simulink library "CreateCovDiagMatrix"  (R2018b)
settings: Solver=VariableStepAuto  StartTime=0.0  StopTime=10.0  RelTol=1e-3
settings Model: Creator=BI28030  LastModifiedBy=BI28030

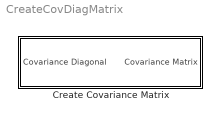
== system CreateCovDiagMatrix ==
  Create Covariance Matrix : Subsystem

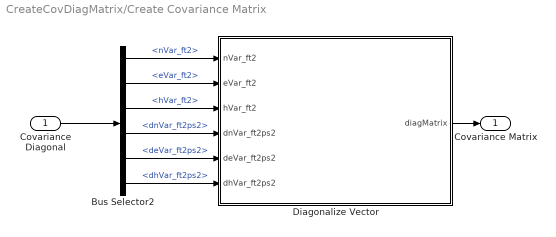
== system CreateCovDiagMatrix/Create Covariance Matrix ==
  Covariance Diagonal : Inport
  Bus Selector2 : BusSelector  OutputSignals=nVar_ft2,eVar_ft2,hVar_ft2,dnVar_ft2ps2,deVar_ft2ps2,dhVar_ft2ps2
  Diagonalize Vector : MATLAB Function  TreatAsAtomicUnit=on
  Covariance Matrix : Outport
  wires:
  Covariance Diagonal/1 -> Bus Selector2/1
  Diagonalize Vector/1(diagMatrix) -> Covariance Matrix/1
  Bus Selector2/1 -> Diagonalize Vector/1(nVar_ft2)  "<nVar_ft2>"
  Bus Selector2/2 -> Diagonalize Vector/2(eVar_ft2)  "<eVar_ft2>"
  Bus Selector2/3 -> Diagonalize Vector/3(hVar_ft2)  "<hVar_ft2>"
  Bus Selector2/4 -> Diagonalize Vector/4(dnVar_ft2ps2)  "<dnVar_ft2ps2>"
  Bus Selector2/5 -> Diagonalize Vector/5(deVar_ft2ps2)  "<deVar_ft2ps2>"
  Bus Selector2/6 -> Diagonalize Vector/6(dhVar_ft2ps2)  "<dhVar_ft2ps2>"

== matlab function CreateCovDiagMatrix/Create Covariance Matrix/Diagonalize Vector ==
  data: nVar_ft2 input; diagMatrix output; eVar_ft2 input; hVar_ft2 input; dnVar_ft2ps2 input; deVar_ft2ps2 input; dhVar_ft2ps2 input
function diagMatrix = createDiagMatrix(nVar_ft2, eVar_ft2, hVar_ft2, dnVar_ft2ps2, deVar_ft2ps2, dhVar_ft2ps2)

diagMatrix = zeros(6);

% diagMatrix(1,1) = diagVector(1);
% diagMatrix(2,2) = diagVector(2);
% diagMatrix(3,3) = diagVector(3);
% diagMatrix(4,4) = diagVector(4);
% diagMatrix(5,5) = diagVector(5);
% diagMatrix(6,6) = diagVector(6);

diagMatrix(1,1) = nVar_ft2;
diagMatrix(2,2) = eVar_ft2;
diagMatrix(3,3) = hVar_ft2;
diagMatrix(4,4) = dnVar_ft2ps2;
diagMatrix(5,5) = deVar_ft2ps2;
diagMatrix(6,6) = dhVar_ft2ps2;
